simulink model "prob2"  (R2015a)
settings: Solver=ode3  StartTime=0.0  StopTime=inf  RelTol=1e-3
settings Model: SimulationMode=external  ExtModeTrigDuration=100  Creator=RafRaeymaekers  LastModifiedBy=RafRaeymaekers
settings OptimizationCC: OptimizeModelRefInitCode=on  LifeSpan=1
settings DebuggingCC: UnderspecifiedInitializationDetection=Classic  MergeDetectMultiDrivingBlocksExec=none
settings HardwareCC: ProdLargestAtomicInteger=Long  ProdLargestAtomicFloat=Double  ProdEndianess=LittleEndian  ProdHWDeviceType=ARM Compatible->ARM Cortex
settings RTWCC: SystemTargetFile=realtime.tlc  GenerateMakefile=off  TemplateMakefile=realtime.tmf  Description=Run on Target Hardware  RTWVerbose=off
settings ERTTargetCC: CombineOutputUpdateFcns=off  ExtModeMexArgs='169.254.0.2' 0 17725  ERTSrcFileBannerTemplate=realtime_code_template.cgt  ERTHdrFileBannerTemplate=realtime_code_template.cgt  ERTDataSrcFileTemplate=realtime_code_template.cgt  ERTDataHdrFileTemplate=realtime_code_template.cgt  ERTCustomFileTemplate=realtime_file_process.tlc

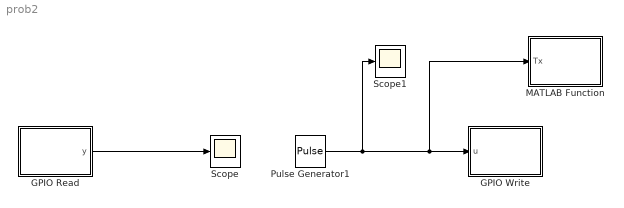
== system prob2 ==
  GPIO Read : MATLAB Function  TreatAsAtomicUnit=on
      settings: CopyFcn=set_param(gcs, 'CustomHeaderCode', '#include <stdio.h>');
  GPIO Write : MATLAB Function  TreatAsAtomicUnit=on
  MATLAB Function : MATLAB Function  TreatAsAtomicUnit=on
  Pulse Generator1 : DiscretePulseGenerator  Period=20  PulseWidth=5  SampleTime=50e-3
  Scope : Scope
  Scope1 : Scope
  wires:
  Pulse Generator1/1 -> Scope1/1, MATLAB Function/1(Tx), GPIO Write/1(u)
  GPIO Read/1(y) -> Scope/1

== matlab function prob2/GPIO Read ==
  data: y output
function y = fcn()
%#codegen

% This MATLAB function shows how to setup and use a GPIO pin as input. The
% function basically issues a number of system calls to do the following:
% 1. Export GPIO pin for use
% 2. Setup GPIO direction as input
% 3. Read GPIO pin logic level and return it in the variable y
% 

persistent firstTime;
persistent pf;
gpioPin = '139';
coder.extrinsic('disp');
if isempty(firstTime)
    firstTime = 0;   
    pf = coder.opaque('FILE *');
    if isequal(coder.target, 'rtw')
        % Export GPIO pin
        cmd1 = c_string(['echo ', gpioPin, '> /sys/class/gpio/export']);
        coder.ceval('system', coder.rref(cmd1));
        % Set GPIO pin direction to output
        cmd2 = c_string(['echo in > /sys/class/gpio/gpio', gpioPin, '/direction']);
        coder.ceval('system', coder.rref(cmd2));
    else
        disp('Initialize GPIO pin as output');
    end
end

% Set GPIO pin logic level using a system call
y = coder.nullcopy(uint8(0));
res = coder.nullcopy(uint8(zeros(1, 10)));
readOnly = c_string('r');
readCmd = c_string(['cat /sys/class/gpio/gpio', gpioPin, '/value']);
if isequal(coder.target, 'rtw')
    pf = coder.ceval('popen', coder.rref(readCmd), coder.rref(readOnly));
    coder.ceval('fgets', coder.wref(res), 10, pf);
    %coder.ceval('printf', c_string('%s\n'), c_string(res));
    if (res(1) == '1')
        y = uint8(1);
    else
        y = uint8(0);
    end
    coder.ceval('pclose', pf);
else
    disp(readCmd);
end

end

function str = c_string(str)
% Convert MATLAB string to C-string by adding a string termination
% character 
str = [str, 0];
end

== matlab function prob2/GPIO Write ==
  data: u input
function fcn(u)
coder.cinclude('<stdio.h>');
%#codegen

% This MATLAB function shows how to setup and use a GPIO pin as output. The
% function basically issues a number of system calls to do the following:
% 1. Export GPIO pin for use
% 2. Setup GPIO direction as output
% 3. Write the value of input signal, u, to the GPIO pin
% 
% Input to this function should be a boolean scalar. If the value of u is positive
% then GPIO pin goes high. Else GPIO pin goes low. 
persistent firstTime;
gpioPin = '15';
coder.extrinsic('disp');
if isempty(firstTime)
    firstTime = 0;
    if isequal(coder.target, 'rtw')
        % Export GPIO pin
        cmd1 = c_string(['echo ', gpioPin, '> /sys/class/gpio/export']);
        coder.ceval('system', coder.rref(cmd1));
        % Set GPIO pin direction to output
        cmd2 = c_string(['echo out> /sys/class/gpio/gpio', gpioPin, '/direction']);
        coder.ceval('system', coder.rref(cmd2));
    else
        disp('Initialize GPIO pin as output');
    end
end

% Set GPIO pin logic level using a system call
if (u > 0)
    cmd = c_string(['echo 1 > /sys/class/gpio/gpio', gpioPin, '/value']);
else
    cmd = c_string(['echo 0 > /sys/class/gpio/gpio', gpioPin, '/value']);
end
if isequal(coder.target, 'rtw')
    coder.ceval('system', coder.rref(cmd));
else
    disp(cmd);
end

end

function str = c_string(str)
% Convert MATLAB string to C-string by adding a string termination
% character 
str = [str, 0];
end

== matlab function prob2/MATLAB Function ==
  data: Tx input
function fcn(Tx)

coder.cinclude('<stdio.h>');
%#codegen
mypi = raspi('169.254.0.2');
myserialdevice = serialdev(mypi,'/dev/ttyAMA0')
write(myserialdevice,Tx,'uint16')
